simulink subsystem "Controls_subsysref"  (R2020a)
settings: Solver=VariableStepAuto  StartTime=0.0  StopTime=10.0  RelTol=1e-3
undefined symbols (not defined in the file): RING_STATUS, TMR
settings Model: Creator=Kiera  LastModifiedBy=Kiera

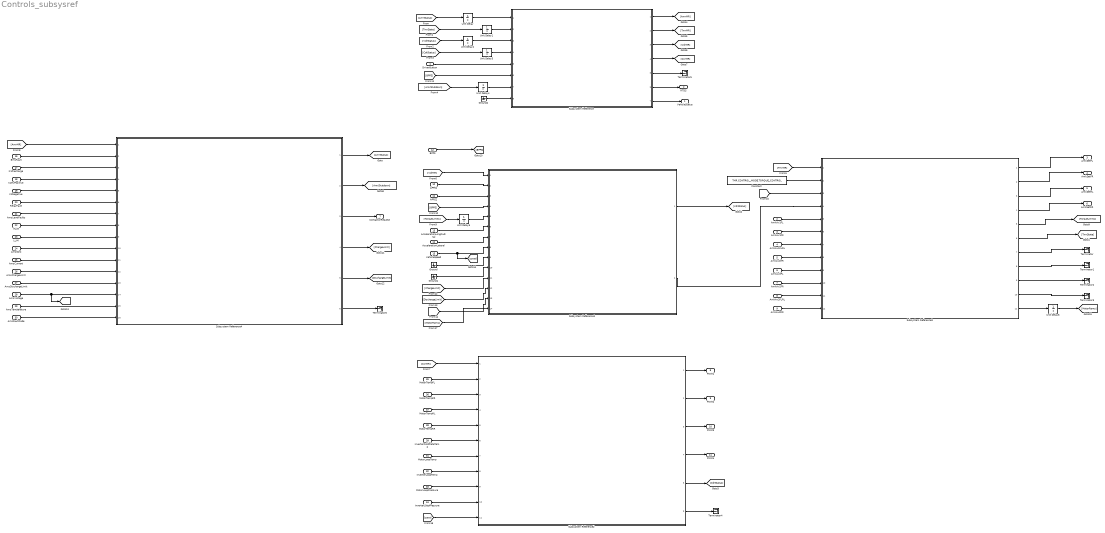
== system Controls_subsysref ==
  DriverButton : Inport  RequirementInfo={} %GIDa_9c594bda_1b0e_4336_8a25_d7f0613eb067
  AmkAv1FL : Inport  RequirementInfo={} %GIDa_fd8c3e23_c3dc_458d_ae3f_8685fb3b1881  Port=2  OutDataTypeStr=Bus: AmkActualValues1
  AmkAv1FR : Inport  RequirementInfo={} %GIDa_308e603c_17d3_43a1_a657_a66bed19ad40  Port=3  OutDataTypeStr=Bus: AmkActualValues1
  AmkAv1FLRL : Inport  RequirementInfo={} %GIDa_d3e0a7e1_5bc0_48ad_8892_cc9d1de443b8  Port=4  OutDataTypeStr=Bus: AmkActualValues1
  AmkAv1RR : Inport  RequirementInfo={} %GIDa_b449e21a_2236_4400_9795_e7cbe8f236da  Port=5  OutDataTypeStr=Bus: AmkActualValues1
  AmkAv2FL : Inport  RequirementInfo={} %GIDa_0b5806f6_aaa7_45f9_9b1a_b4eaf6711fcd  Port=6  OutDataTypeStr=Bus: AmkActualValues2
  AmkAv2FR : Inport  RequirementInfo={} %GIDa_9316be73_f528_47b2_887a_4de99865f183  Port=7  OutDataTypeStr=Bus: AmkActualValues2
  AmkAv2FLRL : Inport  RequirementInfo={} %GIDa_cb97a9a6_b384_472e_9fea_7174b0261c3b  Port=8  OutDataTypeStr=Bus: AmkActualValues2
  AmkAv2RR : Inport  RequirementInfo={} %GIDa_d33f917a_430e_42b4_a23f_af1251bb9c54  Port=9  OutDataTypeStr=Bus: AmkActualValues2
  APPS1 : Inport  RequirementInfo={} %GIDa_23645d8a_cfed_4306_9eb2_2cb720f93fb8  Port=10  OutDataTypeStr=double
  APPS2 : Inport  RequirementInfo={} %GIDa_b7e47a78_e262_42b0_b3fc_a564f2311eac  Port=11  OutDataTypeStr=double
  BPPS : Inport  RequirementInfo={} %GIDa_f1b055d2_f933_4be1_a7ff_ba785610ca74  Port=12  OutDataTypeStr=double
  AccelerationLongitudinal : Inport  RequirementInfo={} %GIDa_d07d1ac4_aab1_4b2d_a049_c821e5e637cf  Port=13  OutDataTypeStr=double
  AccelerationLateral : Inport  RequirementInfo={} %GIDa_370d1226_9ac1_41de_87ea_1415ce68ffbf  Port=14  OutDataTypeStr=double
  VehicleSpeed : Inport  RequirementInfo={} %GIDa_f21d247e_af8c_4023_807a_87da3b66fb31  Port=15
  BmsFault : Inport  RequirementInfo={} %GIDa_e3b68a5c_b691_47d9_9a54_420bf369b197  Port=16
  K1Precharge : Inport  RequirementInfo={} %GIDa_0de62460_c0c3_47c9_b725_6474838c2aa8  Port=17
  K2HvPositive : Inport  RequirementInfo={} %GIDa_4656b82a_a20a_41c6_905a_1668a777f3a5  Port=18
  K3Negative : Inport  RequirementInfo={} %GIDa_bb9301f0_b31d_4587_a7c4_99b6c33eaa56  Port=19
  RelayFault : Inport  RequirementInfo={} %GIDa_9c382b8a_370b_49a0_9660_182c4c0c9750  Port=20
  AmsLevelFaults : Inport  RequirementInfo={} %GIDa_41fb44f2_a7e9_4a1c_9243_4fec44c11c6e  Port=21  OutDataTypeStr=uint8
  HLIM : Inport  RequirementInfo={} %GIDa_465df954_ccf2_4a88_8596_fd2aa63c07cd  Port=22
  LLIM : Inport  RequirementInfo={} %GIDa_0663d8f4_c501_4d6a_a295_786702fc748b  Port=23
  AmsSOC : Inport  RequirementInfo={} %GIDa_bc8ce449_a1e9_461c_a665_23a0ff3c2885  Port=24
  AmsCurrent : Inport  RequirementInfo={} %GIDa_47855b3d_3706_4f50_b68f_9d08dc8213a2  Port=25
  AmsChargeLimit : Inport  RequirementInfo={} %GIDa_87d65a0a_21b0_42fc_8001_7ea47bfc8224  Port=26  OutDataTypeStr=double
  AmsDischargeLimit : Inport  RequirementInfo={} %GIDa_bf00a607_23ca_4861_881b_227fe5563419  Port=27  OutDataTypeStr=double
  AmsVoltage : Inport  RequirementInfo={} %GIDa_7b39dbca_1778_46de_9108_ad78bee863a1  Port=28
  AmsTemperature : Inport  RequirementInfo={} %GIDa_08e82a16_d402_4a91_88c9_d8af834a58be  Port=29
  AmsFaultCode : Inport  RequirementInfo={} %GIDa_37aa41df_483d_484f_b773_c2ac17bff088  Port=30  OutDataTypeStr=uint8
  MotorLoopTemp : Inport  RequirementInfo={} %GIDa_79a2b15f_fbe7_41ee_b3d3_317e1129912b  Port=31
  InverterLoopTemp : Inport  RequirementInfo={} %GIDa_2ad79858_f4ad_4d83_9d34_2f88313a80be  Port=32
  MotorLoopPressure : Inport  RequirementInfo={} %GIDa_36ea27c1_9ef7_4cf1_ab0e_142f61abe15b  Port=33
  InverterLoopPressure : Inport  RequirementInfo={} %GIDa_d7e2b1bd_6bcc_42f9_a62f_237cad429472  Port=34
  MotorTempFL : Inport  RequirementInfo={} %GIDa_610c3c25_67a1_4a25_ba77_3d30388a6e4f  Port=35
  MotorTempFR : Inport  RequirementInfo={} %GIDa_6364db4e_5936_4463_9531_5e69b37f91df  Port=36
  MotorTempRL : Inport  RequirementInfo={} %GIDa_6da912c4_04b5_4433_ab3e_9e7488ef2e14  Port=37
  MotorTempRR : Inport  RequirementInfo={} %GIDa_86173213_396e_4c2c_ace8_c3f56af842cb  Port=38
  InverterColdPlateTemp : Inport  RequirementInfo={} %GIDa_528e4daf_439d_42d0_9cf9_3ef91800b0da  Port=39
  Constant : Constant  RequirementInfo={} %GIDa_8e1fc0bb_1b97_4e78_8f9d_b94329c22a22  Value=TMR.CONTROL_MODE.TORQUE_CONTROL
  Ground : Ground  RequirementInfo={} %GIDa_99034e15_43e5_445d_a5cd_ce0495255661
  Ground1 : Ground  RequirementInfo={} %GIDa_9ad3ebec_b6e8_41f1_8892_02d4f132440c
  Ground2 : Ground  RequirementInfo={} %GIDa_1431000c_0217_49f7_8f70_6153918147d2
  Subsystem Reference : Subsystem  RequirementInfo={} %GIDa_5dc2f430_69b4_4917_8c23_5b527642cf9c  ReferencedSubsystem=ModeSelectionRing_subsysref
  Subsystem Reference1 : Subsystem  RequirementInfo={} %GIDa_f583b4c7_d1b4_4348_9c92_8f39397d0a73  ReferencedSubsystem=VehicleDynamicsRing_subsysref
  Subsystem Reference2 : Subsystem  RequirementInfo={} %GIDa_ed787c48_667f_4511_a044_9b5aa7a7b087  ReferencedSubsystem=CoolingControlRing_subsysref
  Subsystem Reference3 : Subsystem  RequirementInfo={} %GIDa_d0f4cb23_8ab2_46f1_9f3c_eaaa504c147b  ReferencedSubsystem=Tractive_Motor_Ring_Four_Motors_subsysref
  Subsystem Reference4 : Subsystem  RequirementInfo={} %GIDa_355583c4_a0e2_4034_88c7_6418300c9d01  ReferencedSubsystem=AccumulatorManagementRing_subsysref
  Terminator{,1..6} (7 alike) : Terminator
      Terminator settings: RequirementInfo={} %GIDa_64e10c88_f5b2_424f_8df9_1e335281bd0a
      Terminator1 settings: RequirementInfo={} %GIDa_6b4689ab_8b90_4e52_95eb_3539ee560e42
      Terminator2 settings: RequirementInfo={} %GIDa_d650bf7c_72bb_4dc5_80d0_f43b8b259994
      Terminator3 settings: RequirementInfo={} %GIDa_b24eb0e2_9c46_44f1_b538_95e1412717b3
      Terminator4 settings: RequirementInfo={} %GIDa_5f0d96c4_9ea3_4042_bf9a_5aff7daad418
      Terminator5 settings: RequirementInfo={} %GIDa_1d4c48a0_16e9_482e_ac3a_05fdaab52a40
      Terminator6 settings: RequirementInfo={} %GIDa_2c4253c0_2ecc_4061_aa5e_1742d68c6f8f
  Unit Delay : UnitDelay  RequirementInfo={} %GIDa_c7fd52e8_5459_42ed_b2a2_2576ffa386f2  InitialCondition=RING_STATUS.OFF  SampleTime=-1  HasFrameUpgradeWarning=on
  Unit Delay1 : UnitDelay  RequirementInfo={} %GIDa_50a81353_37d6_40d6_ba3b_5abc5d905232  InitialCondition=RING_STATUS.OFF  SampleTime=-1  HasFrameUpgradeWarning=on
  Unit Delay2 : UnitDelay  RequirementInfo={} %GIDa_df296250_7ab2_4d21_8705_8a47680e5dfa  InitialCondition=RING_STATUS.OFF  SampleTime=-1  HasFrameUpgradeWarning=on
  Unit Delay3 : UnitDelay  RequirementInfo={} %GIDa_e39be60d_b5c4_484b_967f_88c379bb63c5  InitialCondition=RING_STATUS.OFF  SampleTime=-1  HasFrameUpgradeWarning=on
  Unit Delay4 : UnitDelay  RequirementInfo={} %GIDa_f14c0532_1c4e_4314_ae8c_fa39b066b2c4  InitialCondition=false  SampleTime=-1  HasFrameUpgradeWarning=on
  Unit Delay5 : UnitDelay  RequirementInfo={} %GIDa_d64cc443_9c52_432a_a0b9_0a8ad0de5f5b  SampleTime=-1  HasFrameUpgradeWarning=on
  Unit Delay6 : UnitDelay  RequirementInfo={} %GIDa_2fb971e0_a7c7_4ad2_a24f_dd9efc796ef1  SampleTime=-1  HasFrameUpgradeWarning=on
  VehicleStatus : Outport  RequirementInfo={} %GIDa_f36d60c3_e6bf_43c3_8807_5baa64c90113  OutDataTypeStr=Enum: VEHICLE_STATUS  VectorParamsAs1DForOutWhenUnconnected=off
  RTDS : Outport  RequirementInfo={} %GIDa_366c1a0e_54c8_4230_9c47_1d982f7a7ed1  Port=2  VectorParamsAs1DForOutWhenUnconnected=off
  AmkSetFL : Outport  RequirementInfo={} %GIDa_bf2bed8b_b0f9_4c24_8abb_ce5390536738  Port=3  OutDataTypeStr=Bus: AmkSetpoints  VectorParamsAs1DForOutWhenUnconnected=off
  AmkSetFR : Outport  RequirementInfo={} %GIDa_334faa22_d445_4449_b1fb_e9278d638fb1  Port=4  OutDataTypeStr=Bus: AmkSetpoints  VectorParamsAs1DForOutWhenUnconnected=off
  AmkSetRL : Outport  RequirementInfo={} %GIDa_11ccc86b_bc0d_46ae_a305_b8f781ea82ed  Port=5  OutDataTypeStr=Bus: AmkSetpoints  VectorParamsAs1DForOutWhenUnconnected=off
  AmkSetRR : Outport  RequirementInfo={} %GIDa_fb20fefc_1026_43f2_af02_edf1f71a3b91  Port=6  OutDataTypeStr=Bus: AmkSetpoints  VectorParamsAs1DForOutWhenUnconnected=off
  ContactorRequest : Outport  RequirementInfo={} %GIDa_6a9d2782_c6f9_4ba3_9dfa_3e94b7616fba  Port=7  VectorParamsAs1DForOutWhenUnconnected=off
  PWM1 : Outport  RequirementInfo={} %GIDa_5b05c93e_6d46_4cff_a7a5_86d42cec9c94  Port=8  VectorParamsAs1DForOutWhenUnconnected=off
  PWM2 : Outport  RequirementInfo={} %GIDa_ce6021a5_0985_4cba_bdab_017fafdca76d  Port=9  VectorParamsAs1DForOutWhenUnconnected=off
  PWM3 : Outport  RequirementInfo={} %GIDa_d916d38f_6e23_4363_ba9a_6b079f8f1dd4  Port=10  VectorParamsAs1DForOutWhenUnconnected=off
  PWM4 : Outport  RequirementInfo={} %GIDa_9637bb45_9c6d_4f4c_9634_a0e16f0cb3f5  Port=11  VectorParamsAs1DForOutWhenUnconnected=off
  wires:
  Subsystem Reference4/4 -> [ChargeLimit]
  Subsystem Reference3/8 -> Terminator1/1
  AmkAv1FL/1 -> Subsystem Reference3/5
  AmkAv1FLRL/1 -> Subsystem Reference3/7
  Constant/1 -> Subsystem Reference3/2
  Subsystem Reference3/5 -> [TorqueLimits]
  Subsystem Reference1/2 -> Subsystem Reference3/4
  [TmrMR] -> Subsystem Reference3/1
  Subsystem Reference3/4 -> AmkSetRR/1
  Subsystem Reference3/3 -> AmkSetRL/1
  Subsystem Reference3/2 -> AmkSetFR/1
  Subsystem Reference3/1 -> AmkSetFL/1
  Subsystem Reference3/6 -> [TmrState]
  AmkAv2FL/1 -> Subsystem Reference3/9
  Subsystem Reference3/9 -> Terminator2/1
  Unit Delay1/1 -> Subsystem Reference/2
  Subsystem Reference/1 -> [AmrMR]
  Unit Delay4/1 -> Subsystem Reference/7
  [BPPS] -> Subsystem Reference/6
  Ground2/1 -> Subsystem Reference/8
  DriverButton/1 -> Subsystem Reference/5
  Subsystem Reference3/11 -> Unit Delay6/1
  [DischargeLimit] -> Subsystem Reference1/12
  Subsystem Reference/4 -> [CcrMR]
  Subsystem Reference/2 -> [TmrMR]
  Unit Delay/1 -> Subsystem Reference/1
  Unit Delay2/1 -> Subsystem Reference/3
  Subsystem Reference/7 -> VehicleStatus/1
  Subsystem Reference/6 -> RTDS/1
  [TorqueLimits] -> Unit Delay5/1
  [AmrStatus] -> Unit Delay/1
  Unit Delay3/1 -> Subsystem Reference/4
  [VdrStatus] -> Unit Delay2/1
  Subsystem Reference4/6 -> Terminator6/1
  Subsystem Reference4/1 -> [AmrStatus]
  AmsFaultCode/1 -> Subsystem Reference4/16
  Subsystem Reference4/2 -> [AmrShutdown]
  HLIM/1 -> Subsystem Reference4/8
  [AmrShutdown] -> Unit Delay4/1
  AmsDischargeLimit/1 -> Subsystem Reference4/13
  [CdrStatus] -> Unit Delay3/1
  Subsystem Reference1/1 -> [VdrStatus]
  RelayFault/1 -> Subsystem Reference4/6
  [MotorRpms] -> Subsystem Reference1/14
  Subsystem Reference/5 -> Terminator5/1
  AmkAv1FR/1 -> Subsystem Reference3/6
  [AmrMR] -> Subsystem Reference4/1
  BmsFault/1 -> Subsystem Reference4/2
  [VdrMR] -> Subsystem Reference1/1
  K1Precharge/1 -> Subsystem Reference4/3
  AmsChargeLimit/1 -> Subsystem Reference4/12
  [TmrState] -> Unit Delay1/1
  AmkAv2FLRL/1 -> Subsystem Reference3/11
  AmkAv2RR/1 -> Subsystem Reference3/12
  MotorLoopPressure/1 -> Subsystem Reference2/9
  AmsTemperature/1 -> Subsystem Reference4/15
  InverterLoopPressure/1 -> Subsystem Reference2/10
  MotorLoopTemp/1 -> Subsystem Reference2/7
  InverterColdPlateTemp/1 -> Subsystem Reference2/6
  K2HvPositive/1 -> Subsystem Reference4/4
  [Voltage] -> Subsystem Reference3/3
  MotorTempRR/1 -> Subsystem Reference2/5
  MotorTempFL/1 -> Subsystem Reference2/2
  [Voltage] -> Subsystem Reference1/13
  AccelerationLateral/1 -> Subsystem Reference1/7
  AccelerationLongitudinal/1 -> Subsystem Reference1/6
  LLIM/1 -> Subsystem Reference4/9
  AmkAv1RR/1 -> Subsystem Reference3/8
  Subsystem Reference4/5 -> [DischargeLimit]
  [BPPS] -> Subsystem Reference1/4
  K3Negative/1 -> Subsystem Reference4/5
  Subsystem Reference3/10 -> Terminator3/1
  APPS1/1 -> Subsystem Reference1/2
  APPS2/1 -> Subsystem Reference1/3
  AmsSOC/1 -> Subsystem Reference4/10
  [ChargeLimit] -> Subsystem Reference1/11
  AmsLevelFaults/1 -> Subsystem Reference4/7
  Ground1/1 -> Subsystem Reference1/10
  Subsystem Reference2/6 -> Terminator4/1
  Subsystem Reference3/7 -> Terminator/1
  MotorTempRL/1 -> Subsystem Reference2/4
  Subsystem Reference2/5 -> [CdrStatus]
  Unit Delay5/1 -> Subsystem Reference1/5
  [CcrMR] -> Subsystem Reference2/1
  InverterLoopTemp/1 -> Subsystem Reference2/8
  Subsystem Reference2/3 -> PWM3/1
  Subsystem Reference2/4 -> PWM4/1
  Subsystem Reference/3 -> [VdrMR]
  Ground/1 -> Subsystem Reference1/9
  Subsystem Reference4/3 -> ContactorRequest/1
  Subsystem Reference2/1 -> PWM1/1
  Unit Delay6/1 -> [MotorRpms]
  AmsVoltage/1 -> Subsystem Reference4/14, [Voltage]
  Subsystem Reference2/2 -> PWM2/1
  MotorTempFR/1 -> Subsystem Reference2/3
  BPPS/1 -> [BPPS]
  VehicleSpeed/1 -> Subsystem Reference1/8, [speed]
  AmkAv2FR/1 -> Subsystem Reference3/10
  AmsCurrent/1 -> Subsystem Reference4/11
  [speed] -> Subsystem Reference2/11
